simulink model "test_VisionModel"  (Simulink 7.6)
settings: Solver=FixedStepDiscrete  StartTime=0.0  StopTime=0  RelTol=1e-3
values from neighbouring files (symbols this model uses):
  black_al = 0    [VisionConstants.m]
  black_au = 0    [VisionConstants.m]
  black_bl = 0    [VisionConstants.m]
  black_bu = 0    [VisionConstants.m]
  blue_al = 0    [VisionConstants.m]
  blue_au = 0    [VisionConstants.m]
  blue_bl = 0    [VisionConstants.m]
  blue_bu = 0    [VisionConstants.m]
  green_al = -128    [VisionConstants.m]
  green_au = -25    [VisionConstants.m]
  green_bl = -5    [VisionConstants.m]
  green_bu = 127    [VisionConstants.m]
  orange_al = 5    [VisionConstants.m]
  orange_au = 10    [VisionConstants.m]
  orange_bl = 30    [VisionConstants.m]
  orange_bu = 34    [VisionConstants.m]
  red_al = 25    [VisionConstants.m]
  red_au = 127    [VisionConstants.m]
  red_bl = 0    [VisionConstants.m]
  red_bu = 127    [VisionConstants.m]
  white_al = 0    [VisionConstants.m]
  white_au = 0    [VisionConstants.m]
  white_bl = 0    [VisionConstants.m]
  white_bu = 0    [VisionConstants.m]
  yellow_al = 0    [VisionConstants.m]
  yellow_au = 0    [VisionConstants.m]
  yellow_bl = 0    [VisionConstants.m]
  yellow_bu = 0    [VisionConstants.m]
undefined symbols (not defined in the file or in its folder): gray
libraries: vipsnks x2, vipsrcs x2
settings Model: Creator=Thing 1  LastModifiedBy=auvt
settings OptimizationCC: InlineParams=on  OptimizeModelRefInitCode=on
settings RTWCC: SystemTargetFile=ert.tlc  GenCodeOnly=on  TemplateMakefile=ert_default_tmf  Description=Real-Time Workshop Embedded Coder  GenerateReport=on  ProcessScript=ert_make_rtw_hook  IncludeHyperlinkInReport=on  LaunchReport=on  TargetLang=C++
settings CodeAppCC: IgnoreCustomStorageClasses=off
settings ERTTargetCC: MultiwordLength=2048  GenerateSampleERTMain=on  IncludeMdlTerminateFcn=off  ERTCustomFileTemplate=example_file_process.tlc  ConvertIfToSwitch=off

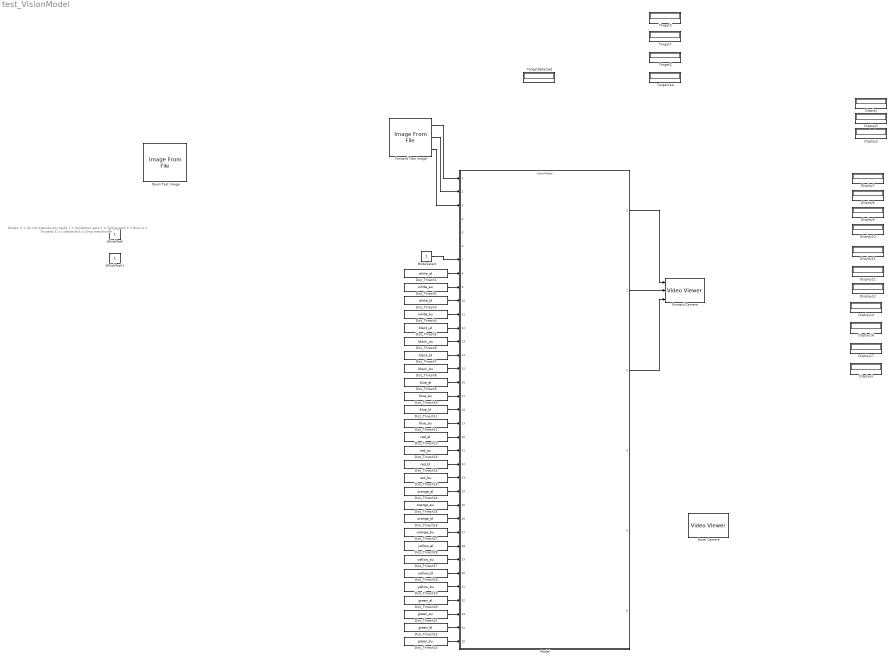
== system test_VisionModel ==
  note: Modes:
      | 0 = Do not execute any tasks
      | 1 = Validation gate
      | 2 = Follow path
      | 3 = Buoy
      | 4 = Torpedo
      | 5 = L-obstacle
      | 6 = Drop mecahnism
  Display{,1..3,7..14,16..17} (14 alike) : Display
  Dist_Thresh1 : Constant  Value=white_al  SampleTime=-1
  Dist_Thresh10 : Constant  Value=blue_au  SampleTime=-1
  Dist_Thresh11 : Constant  Value=blue_bl  SampleTime=-1
  Dist_Thresh12 : Constant  Value=blue_bu  SampleTime=-1
  Dist_Thresh13 : Constant  Value=red_al  SampleTime=-1
  Dist_Thresh14 : Constant  Value=red_au  SampleTime=-1
  Dist_Thresh15 : Constant  Value=red_bl  SampleTime=-1
  Dist_Thresh16 : Constant  Value=red_bu  SampleTime=-1
  Dist_Thresh17 : Constant  Value=yellow_au  SampleTime=-1
  Dist_Thresh18 : Constant  Value=yellow_bl  SampleTime=-1
  Dist_Thresh19 : Constant  Value=yellow_bu  SampleTime=-1
  Dist_Thresh2 : Constant  Value=white_au  SampleTime=-1
  Dist_Thresh20 : Constant  Value=green_al  SampleTime=-1
  Dist_Thresh21 : Constant  Value=green_au  SampleTime=-1
  Dist_Thresh22 : Constant  Value=green_bl  SampleTime=-1
  Dist_Thresh23 : Constant  Value=green_bu  SampleTime=-1
  Dist_Thresh24 : Constant  Value=orange_al  SampleTime=-1
  Dist_Thresh25 : Constant  Value=orange_au  SampleTime=-1
  Dist_Thresh26 : Constant  Value=orange_bl  SampleTime=-1
  Dist_Thresh27 : Constant  Value=orange_bu  SampleTime=-1
  Dist_Thresh28 : Constant  Value=yellow_al  SampleTime=-1
  Dist_Thresh3 : Constant  Value=white_bl  SampleTime=-1
  Dist_Thresh4 : Constant  Value=white_bu  SampleTime=-1
  Dist_Thresh5 : Constant  Value=black_al  SampleTime=-1
  Dist_Thresh6 : Constant  Value=black_au  SampleTime=-1
  Dist_Thresh7 : Constant  Value=black_bl  SampleTime=-1
  Dist_Thresh8 : Constant  Value=black_bu  SampleTime=-1
  Dist_Thresh9 : Constant  Value=blue_al  SampleTime=-1
  Down Camera : vipsnks/Video Viewer  DialogControllerArgs=DataTag1  inputType=Obsolete7b  imagePorts=Separate color signals  useColorMap=off  colormapValue=gray(256)  specRange=off  minInputVal=0  maxInputVal=255  FigPos=[2606 839 364 553]  AxisZoom=on  trueSizedOnce=off  OpenAtMdlStart=on
  Down Test Image : vipsrcs/Image From File  Tag=vipblks_nd  DialogController=vipDDGCreate  DialogControllerArgs=DataTag2  SystemSampleTime=-1  FileName=/home/auvt/auvc/src/vision/Test_Images/path10.bmp  imagePorts=Separate color signals  Ts=-1  ImageDataType=double  Signed=on  WordLength=16  sdImageDataType=uint(8)  FractionLengthMode=User-defined  FractionLength=15  OutPortLabels=R|G|B
  Forward Camera : vipsnks/Video Viewer  DialogControllerArgs=DataTag4  inputType=Obsolete7b  imagePorts=Separate color signals  useColorMap=off  colormapValue=gray(256)  specRange=off  minInputVal=0  maxInputVal=255  FigPos=[1039 758 364 553]  AxisZoom=on  trueSizedOnce=off  OpenAtMdlStart=on
  Forward Test Image : vipsrcs/Image From File  Tag=vipblks_nd  DialogController=vipDDGCreate  DialogControllerArgs=DataTag5  SystemSampleTime=-1  FileName=/home/auvt/auvc/src/vision/Test_Images/gate14.bmp  imagePorts=Separate color signals  Ts=-1  ImageDataType=double  Signed=on  WordLength=16  sdImageDataType=uint(8)  FractionLengthMode=User-defined  FractionLength=15  OutPortLabels=R|G|B
  ModeSelect : Constant  SampleTime=-1
  Model : ModelReference  ModelNameDialog=VisionModel  SimulationMode=Accelerator  ModelReferenceVersion=1.751  CopyOfModelName=VisionModel
  TargetDetected : Display
  TargetX : Display
  TargetY : Display
  TargetYaw : Display
  TargetZ : Display
  WhichPath : Constant  SampleTime=-1
  WhichPath1 : Constant  SampleTime=-1
  wires:
  Forward Test Image/1 -> Model/1
  Forward Test Image/2 -> Model/2
  Forward Test Image/3 -> Model/3
  Dist_Thresh1/1 -> Model/8
  Dist_Thresh23/1 -> Model/35
  Dist_Thresh2/1 -> Model/9
  Dist_Thresh3/1 -> Model/10
  Dist_Thresh4/1 -> Model/11
  Dist_Thresh5/1 -> Model/12
  Dist_Thresh6/1 -> Model/13
  Dist_Thresh7/1 -> Model/14
  Dist_Thresh8/1 -> Model/15
  Dist_Thresh9/1 -> Model/16
  Dist_Thresh10/1 -> Model/17
  Dist_Thresh11/1 -> Model/18
  Dist_Thresh12/1 -> Model/19
  Dist_Thresh13/1 -> Model/20
  Dist_Thresh14/1 -> Model/21
  Dist_Thresh15/1 -> Model/22
  Dist_Thresh16/1 -> Model/23
  Dist_Thresh24/1 -> Model/24
  Dist_Thresh25/1 -> Model/25
  Dist_Thresh26/1 -> Model/26
  Dist_Thresh27/1 -> Model/27
  Dist_Thresh28/1 -> Model/28
  Dist_Thresh17/1 -> Model/29
  Dist_Thresh18/1 -> Model/30
  Dist_Thresh19/1 -> Model/31
  Dist_Thresh20/1 -> Model/32
  Dist_Thresh21/1 -> Model/33
  Dist_Thresh22/1 -> Model/34
  Model/3 -> Forward Camera/3
  Model/2 -> Forward Camera/2
  Model/1 -> Forward Camera/1
  ModeSelect/1 -> Model/7
